simulink model "CrCLmp_DD"  (R2016b)
settings: configuration reference "CodeGenConfigSet" (kept outside this file)
values from neighbouring files (symbols this model uses):
  CrCLmp_stPsDiaDisblSet_C = Calibration.Parameter    [init_CrCLmp_DD.m]
  CrCLmp_stPsDisblSet_C = Calibration.Parameter    [init_CrCLmp_DD.m]
libraries: simulink x2
settings Model: Creator=xinchangran  LastModifiedBy=xinchangran
settings ConfigSetRef: SourceLocation=Base Workspace

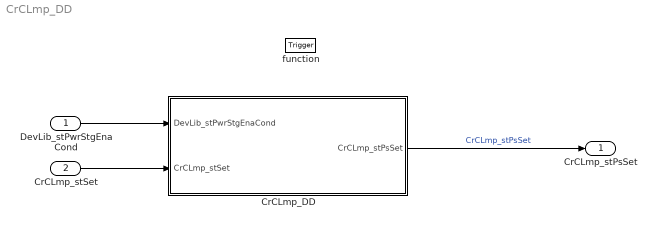
== system CrCLmp_DD ==
  DevLib_stPwrStgEnaCond : Inport  Description=Control unit status relevant to power stage deactivation/error diagnosis  OutMin=0  OutMax=65535  OutDataTypeStr=State_uint16
  CrCLmp_stSet : Inport  Description=input from ASW for cruise set lamp ON/OFF  Port=2  OutMin=0  OutMax=1  OutDataTypeStr=boolean
  function : TriggerPort  TriggerType=function-call  VariantControl=Variant
  CrCLmp_DD : Subsystem
  CrCLmp_stPsSet : Outport  Description=digital output ON/OFF control for set lamp  OutMin=0  OutMax=1  OutDataTypeStr=boolean
  wires:
  DevLib_stPwrStgEnaCond/1 -> CrCLmp_DD/1(DevLib_stPwrStgEnaCond)
  CrCLmp_stSet/1 -> CrCLmp_DD/2(CrCLmp_stSet)
  CrCLmp_DD/1(CrCLmp_stPsSet) -> CrCLmp_stPsSet/1  "CrCLmp_stPsSet"

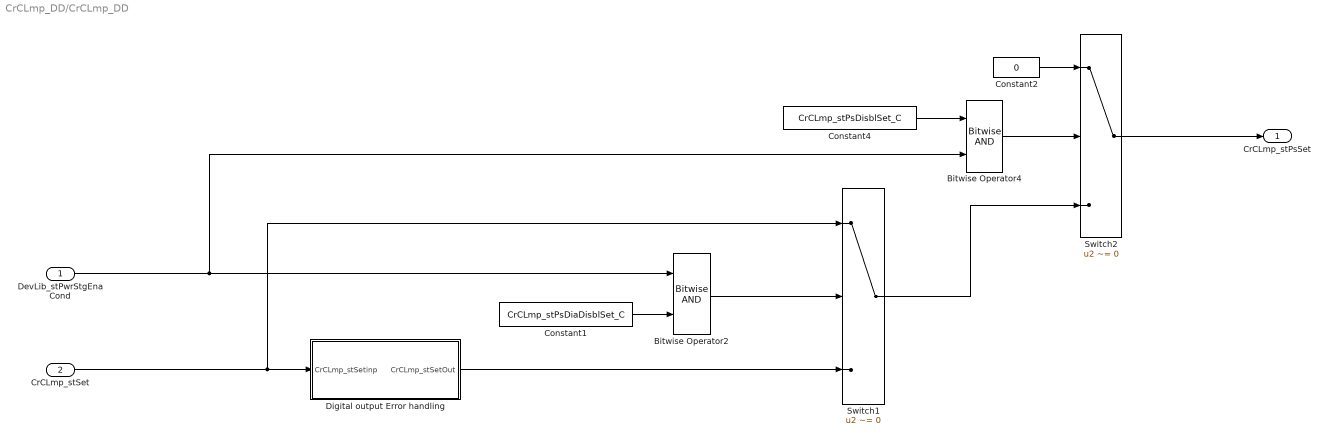
== system CrCLmp_DD/CrCLmp_DD ==
  DevLib_stPwrStgEnaCond : Inport  Description=Control unit status relevant to power stage deactivation/error diagnosis  OutMin=0  OutMax=65535  OutDataTypeStr=State_uint16
  CrCLmp_stSet : Inport  Description=input from ASW for cruise set lamp ON/OFF  Port=2  OutMin=0  OutMax=1  OutDataTypeStr=boolean
  Bitwise Operator2 : simulink/Logic and Bit Operations/Bitwise Operator  logicop=AND  UseBitMask=off  NumInputPorts=2  BitMask=bin2dec('00010000')  BitMaskRealWorld=Stored Integer
  Bitwise Operator4 : simulink/Logic and Bit Operations/Bitwise Operator  logicop=AND  UseBitMask=off  NumInputPorts=2  BitMask=bin2dec('00010000')  BitMaskRealWorld=Stored Integer
  Constant1 : Constant  Value=CrCLmp_stPsDiaDisblSet_C
  Constant2 : Constant  Value=0  OutDataTypeStr=Inherit: Inherit via back propagation
  Constant4 : Constant  Value=CrCLmp_stPsDisblSet_C
  Digital output Error handling : Subsystem
  Switch1 : Switch  Criteria=u2 ~= 0  SaturateOnIntegerOverflow=on  InputSameDT=on
  Switch2 : Switch  Criteria=u2 ~= 0  SaturateOnIntegerOverflow=on  InputSameDT=on
  CrCLmp_stPsSet : Outport  Description=digital output ON/OFF control for set lamp  OutMin=0  OutMax=1  OutDataTypeStr=boolean
  wires:
  CrCLmp_stSet/1 -> Switch1/1, Digital output Error handling/1(CrCLmp_stSetinp)
  Switch2/1 -> CrCLmp_stPsSet/1
  Switch1/1 -> Switch2/3
  Bitwise Operator4/1 -> Switch2/2
  DevLib_stPwrStgEnaCond/1 -> Bitwise Operator4/2, Bitwise Operator2/1
  Digital output Error handling/1(CrCLmp_stSetOut) -> Switch1/3
  Constant4/1 -> Bitwise Operator4/1
  Bitwise Operator2/1 -> Switch1/2
  Constant1/1 -> Bitwise Operator2/2
  Constant2/1 -> Switch2/1

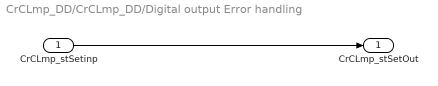
== system CrCLmp_DD/CrCLmp_DD/Digital output Error handling ==
  CrCLmp_stSetinp : Inport
  CrCLmp_stSetOut : Outport
  wires:
  CrCLmp_stSetinp/1 -> CrCLmp_stSetOut/1
